simulink model "controllo_disco_rigido_final"  (R2019b)
settings: Solver=VariableStepAuto  StartTime=0.0  StopTime=10  FixedStep=0.01  RelTol=1e-3
values from neighbouring files (symbols this model uses):
  b = 0.002    [controllo_disco_rigido.m]    (also in controllo_disco_rigido_baseWS.mat; controllo_disco_rigido_script.m; init_controllo_disco_rigido.m)
  delay = 0.3    [controllo_disco_rigido.m]    (also in controllo_disco_rigido_script.m)
  J = 0.001    [controllo_disco_rigido.m]    (also in controllo_disco_rigido_baseWS.mat; controllo_disco_rigido_script.m; init_controllo_disco_rigido.m)
  P_den = 10^4*[1 2]    [controllo_disco_rigido.m]
  P_num = [1500 19600]    [controllo_disco_rigido.m]
  R1_n = 10000    [controllo_disco_rigido.m]    (also in controllo_disco_rigido_script.m = 35000)
  R2_n_den = [1 1540 196000]    [controllo_disco_rigido.m]
  R2_n_num = [1 2]    [controllo_disco_rigido.m]
settings Model: Creator=Utente  LastModifiedBy=Utente
settings DataIOCC: ReturnWorkspaceOutputsName=MdlFnl

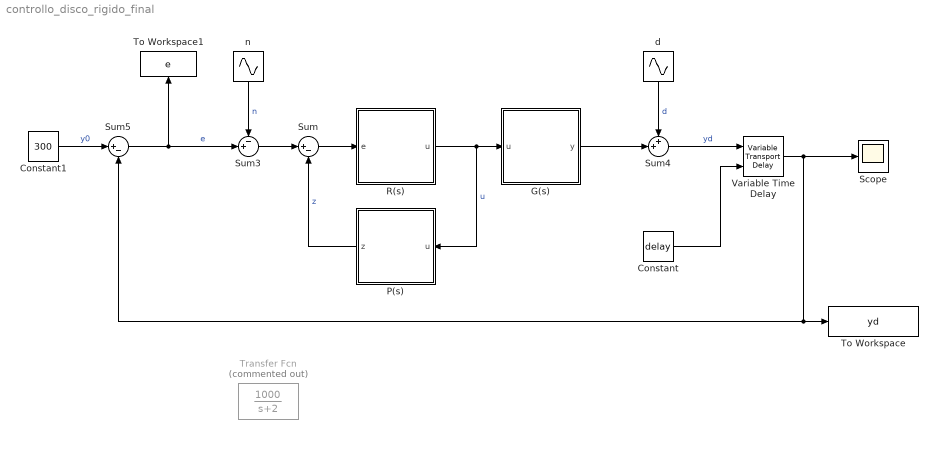
== system controllo_disco_rigido_final ==
  Constant : Constant  Value=delay
  Constant1 : Constant  Value=300
  G(s) : Subsystem
  P(s) : Subsystem
  R(s) : Subsystem
  Scope : Scope
  Sum : Sum  Inputs=|+-
  Sum3 : Sum  Inputs=-+|
  Sum4 : Sum  Inputs=++|
  Sum5 : Sum  Inputs=|+-
  To Workspace : ToWorkspace  VariableName=yd  SampleTime=-1
  To Workspace1 : ToWorkspace  VariableName=e  SampleTime=-1
  Transfer Fcn : TransferFcn  Commented=on  Numerator=[1000]  Denominator=[1 2]
  Variable Time Delay : VariableTransportDelay  MaximumDelay=delay
  d : Sin  Frequency=[5]  SampleTime=0
  n : Sin  Frequency=[50]  SampleTime=0
  wires:
  n/1 -> Sum3/1  "n"
  Sum5/1 -> Sum3/2, To Workspace1/1  "e"
  d/1 -> Sum4/1  "d"
  Constant1/1 -> Sum5/1  "y0"
  R(s)/1(u) -> P(s)/1(u), G(s)/1(u)  "u"
  G(s)/1(y) -> Sum4/2
  Constant/1 -> Variable Time Delay/2
  Variable Time Delay/1 -> Sum5/2, To Workspace/1, Scope/1
  Sum4/1 -> Variable Time Delay/1  "yd"
  Sum3/1 -> Sum/1
  Sum/1 -> R(s)/1(e)
  P(s)/1(z) -> Sum/2  "z"

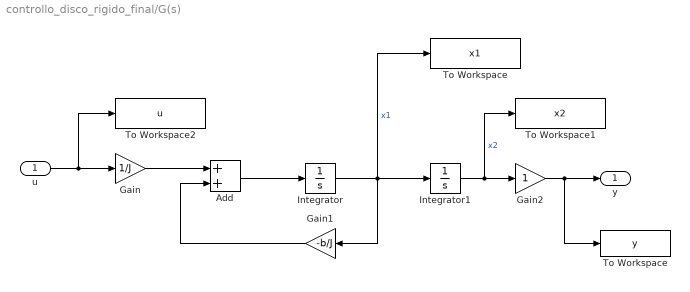
== system controllo_disco_rigido_final/G(s) ==
  u : Inport
  " To Workspace" : ToWorkspace  VariableName=y  SampleTime=-1
  Add : Sum
  Gain : Gain  Gain=1/J
  Gain1 : Gain  Gain=-b/J
  Gain2 : Gain
  Integrator : Integrator
  Integrator1 : Integrator
  To Workspace : ToWorkspace  VariableName=x1  SampleTime=-1
  To Workspace1 : ToWorkspace  VariableName=x2  SampleTime=-1
  To Workspace2 : ToWorkspace  VariableName=u  SampleTime=-1
  y : Outport
  wires:
  Integrator/1 -> To Workspace/1, Gain1/1, Integrator1/1  "x1"
  u/1 -> Gain/1, To Workspace2/1
  Add/1 -> Integrator/1
  Gain/1 -> Add/1
  Gain1/1 -> Add/2
  Integrator1/1 -> Gain2/1, To Workspace1/1  "x2"
  Gain2/1 -> " To Workspace"/1, y/1

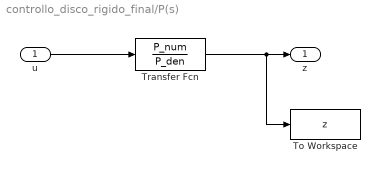
== system controllo_disco_rigido_final/P(s) ==
  u : Inport
  To Workspace : ToWorkspace  VariableName=z  SampleTime=-1
  Transfer Fcn : TransferFcn  Numerator=P_num  Denominator=P_den
  z : Outport
  wires:
  Transfer Fcn/1 -> z/1, To Workspace/1
  u/1 -> Transfer Fcn/1

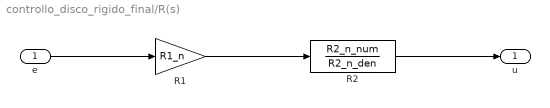
== system controllo_disco_rigido_final/R(s) ==
  e : Inport
  R1 : Gain  Gain=R1_n
  R2 : TransferFcn  Numerator=R2_n_num  Denominator=R2_n_den
  u : Outport
  wires:
  R2/1 -> u/1
  R1/1 -> R2/1
  e/1 -> R1/1
